simulink model "untitled"  (R2019b)
settings: Solver=VariableStepAuto  StartTime=0.0  StopTime=300  FixedStep=0.01  RelTol=1e-3
undefined symbols (not defined in the file): alpha1, alpha2, beta1, beta2, CaCO2_IC, CaO2_IC, Cbp, Cbv, Cep, Cev, Chp, Chv, Cla, Cmp, Cmv, Cpa, Cpp, Cps, Cpv, Cra, Csa, CsatCO2, CsatO2, Csp, Csv, CvCO2_IC, CvO2_IC, D1, D2, Dc, Dp, dt, Emaxlv, Emaxrv, f, fac_max, fac_min, facn, FICO2, FIO2, GcA, Gcf, GpA, Gpf, h1, h2, HR, K1, K1_tv, K2, K2_tv, kac, kElv, kErv, KH, KR, kRlv, kRrv, ksys, Kxp ... (+70)
libraries: fl_lib x42, nesl_utility x9, powerlib_meascontrol x1
(part 2 of 2)

== matlab function untitled/Subsystem5/MATLAB Function ==
  data: PaCO2 input; fac output; PaO2 input; KH parameter; fac_max parameter; fac_min parameter; PO2ac parameter; kac parameter; PaCO2n parameter; f parameter; dt parameter; Tau_ac parameter
function fac  = fnc(PaCO2, PaO2, KH, fac_max, fac_min, PO2ac, kac, PaCO2n, f, dt, Tau_ac)
persistent fac_1;
if isempty(fac_1)
    fac_1 = 3.7;  
end

% B.4.2
if PaO2 >= 80
    K = KH;
elseif 80 >= PaO2 >= 40
    K = KH - 1.2*(PaO2-80)/30;
else
    K = KH - 1.6;
% B.4.1   
Phiac=((fac_max + fac_min*exp((PaO2-PO2ac)/kac)) / 1+ exp((PaO2-PO2ac)/kac)) * (K*log(PaCO2/PaCO2n)+f);


RHS = (Phiac - fac_1)/ Tau_ac;
fac = fac_1 + dt*RHS;

fac_1 = fac;
end
